simulink model "ARSinit"  (Simulink 6.6)
settings: Solver=ode1  SolverMode=SingleTasking  StartTime=0.0  StopTime=Tsim  FixedStep=0.001  RelTol=1e-3
PreLoadFcn:
  | load ARSdata
values from neighbouring files (symbols this model uses):
  car =     [ARSdata.mat]
  K = 0.025    [ARSdata.mat]
  meled_den = [1 -0.980198019802]    [ARSdata.mat]
  meled_num = [0.0049504950495 0.0049504950495]    [ARSdata.mat]
  mmecd_den = [1 -1]    [ARSdata.mat]
  mmecd_num = [0.05 0.05]    [ARSdata.mat]
  phid_den = [1 -1]    [ARSdata.mat]
  phid_num = [0.0005 0.0005]    [ARSdata.mat]
  scrtd_den = [1 -0.818181818182]    [ARSdata.mat]
  scrtd_num = [0.0181818181818 0.0181818181818]    [ARSdata.mat]
  sspeedd_den = [1 -0.818181818182]    [ARSdata.mat]
  sspeedd_num = [0.00909090909091 0.00909090909091]    [ARSdata.mat]
  vconvd_den = [1 -0.818181818182]    [ARSdata.mat]
  vconvd_num = [0.0909090909091 0.0909090909091]    [ARSdata.mat]
undefined symbols (not defined in the file or in its folder): sigbuilder_block
libraries: cstblocks x1
CloseFcn:
  | rtwprivate ssgencode ModelCloseRequest ARSinit
settings Model: Creator=Magna Steyr and PreeTec  LastModifiedBy=derler  ExtModeAutoUpdateStatusClock=off
settings OptimizationCC: InlineInvariantSignals=on  OptimizeModelRefInitCode=on  LifeSpan=1
settings DebuggingCC: SignalResolutionControl=TryResolveAllWithWarning  MultiTaskDSMMsg=warning  MultiTaskCondExecSysMsg=none  StrictBusMsg=None
settings RTWCC: SystemTargetFile=ert.tlc  GenCodeOnly=on  TemplateMakefile=ert_default_tmf  Description=RTW Embedded Coder (no auto configuration)  ProcessScript=ert_make_rtw_hook  IncludeERTFirstTime=on
settings CodeAppCC: IgnoreCustomStorageClasses=off
settings ERTTargetCC: TargetFcnLib=ansi_tfl_tmw.mat  GenFloatMathFcnCalls=ANSI_C  GenerateSampleERTMain=on  SupportContinuousTime=on  SupportNonInlinedSFcns=on  InlinedParameterPlacement=NonHierarchical  ERTCustomFileTemplate=example_file_process.tlc

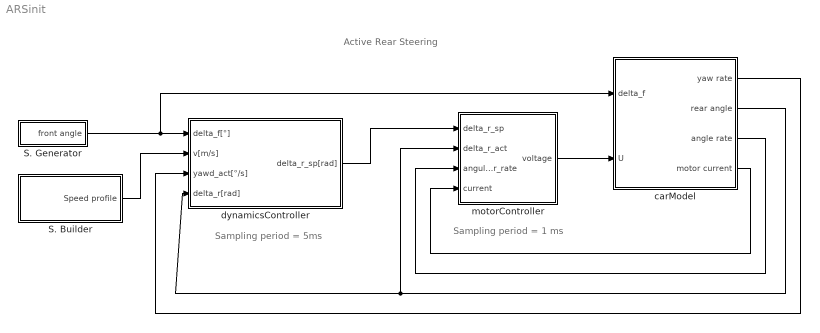
== system ARSinit ==
  note: Sampling period = 5ms
  note: Sampling period = 1 ms
  note: Active Rear Steering
  S. Builder : Subsystem  Tag=STV Subsys  LoadFcn=sigbuilder_block('load',[207 158.25 519.75 399.75 ]);  StartFcn=sigbuilder_block('start');  StopFcn=sigbuilder_block('stop');  ClipboardFcn=sigbuilder_block('clipboard');  mask(Sigbuilder block){}
      mask help: Sigbuilder GUI
      mask init:
      | if ~strcmp(get_param(bdroot(gcbh),'SimulationStatus'),'stopped') tuvar = sigbuilder_block('maskInit'); end
      settings: CopyFcn=sigbuilder_block('copy');  DeleteFcn=sigbuilder_block('delete');  ModelCloseFcn=sigbuilder_block('modelClose');  PreSaveFcn=sigbuilder_block('preSave');  NameChangeFcn=sigbuilder_block('namechange');  OpenFcn=sigbuilder_block('open',[207 158.25 519.75 399.75 ]);  CloseFcn=sigbuilder_block('close');
      mask Display: plot(0,0,100,100,[10,10,40,40,10],[80,20,20,80,80],[40,10],[50,50], [40,27,10],[65,72,56],[40,25,25,10],[28,28,43,43]);
  S. Generator : Subsystem
  carModel : Subsystem  TreatAsAtomicUnit=on  SystemSampleTime=0.001  RTWFcnName=carModel
      settings: RTWSystemCode=Function  RTWFcnNameOpts=User specified  RTWFileNameOpts=Use function name
  dynamicsController : Subsystem  TreatAsAtomicUnit=on  SystemSampleTime=0.005  RTWFcnName=dynamicsController
      settings: RTWSystemCode=Function  RTWFcnNameOpts=User specified  RTWFileNameOpts=Use function name
  motorController : Subsystem  TreatAsAtomicUnit=on  SystemSampleTime=0.001  RTWFcnName=motorController
      settings: RTWSystemCode=Function  RTWFcnNameOpts=User specified  RTWFileNameOpts=Use function name
  wires:
  S. Generator/1(front angle) -> dynamicsController/1(delta_f[°]), carModel/1(delta_f)
  S. Builder/1(Speed profile) -> dynamicsController/2(v[m/s])
  carModel/4(motor current) -> motorController/4(current)
  carModel/3(angle rate) -> motorController/3(angular_rate)
  carModel/2(rear angle) -> motorController/2(delta_r_act), dynamicsController/4(delta_r[rad])
  motorController/1(voltage) -> carModel/2(U)
  dynamicsController/1(delta_r_sp[rad]) -> motorController/1(delta_r_sp)
  carModel/1(yaw rate) -> dynamicsController/3(yawd_act[°/s])

== system ARSinit/S. Builder ==
  Demux : Demux  Tag=STV Demux  Outputs=1
  FromWs : FromWorkspace  Tag=STV FromWs  VariableName=tuvar  SampleTime=0.001  OutputAfterFinalValue=Holding final value  SigBuilderData=DataTag0  VnvData=DataTag1
      SigBuilderData=|
      | channels.label = 'Speed profile'
      | channels.allXData = {[0 8 11 20]}
      | channels.allYData = {[1.4 1.4 13.4 13.4]}
      | dataSet.timeRange = [0 20]
      | dataSet.name = 'Group 1'
  Speed profile : Outport  Tag=STV Outport
  wires:
  Demux/1 -> Speed profile/1
  FromWs/1 -> Demux/1

== system ARSinit/S. Generator ==
  Sum : Sum  Inputs=|++++
  smooth jump1 : Subsystem  AncestorBlock=joeslibrary/smooth jump  mask(Smooth jump){jump_time=6, minimum=-60, maximum=0, k=-10}
      mask prompts: jump_time "Jump time:"; minimum "Minimum value:"; maximum "Maximum value:"; k "Raise value:"
      mask help: x = scaling*tanh(clock-jump_time)
      mask Display: plot(-10:1:10,tanh(-10:1:10))
  smooth jump2 : Subsystem  AncestorBlock=joeslibrary/smooth jump  mask(Smooth jump){jump_time=1, minimum=0, maximum=60, k=10}
      mask prompts: jump_time "Jump time:"; minimum "Minimum value:"; maximum "Maximum value:"; k "Raise value:"
      mask help: x = scaling*tanh(clock-jump_time)
      mask Display: plot(-10:1:10,tanh(-10:1:10))
  smooth jump3 : Subsystem  AncestorBlock=joeslibrary/smooth jump  mask(Smooth jump){jump_time=12, minimum=0, maximum=20, k=10}
      mask prompts: jump_time "Jump time:"; minimum "Minimum value:"; maximum "Maximum value:"; k "Raise value:"
      mask help: x = scaling*tanh(clock-jump_time)
      mask Display: plot(-10:1:10,tanh(-10:1:10))
  smooth jump4 : Subsystem  AncestorBlock=joeslibrary/smooth jump  mask(Smooth jump){jump_time=17, minimum=-20, maximum=0, k=-10}
      mask prompts: jump_time "Jump time:"; minimum "Minimum value:"; maximum "Maximum value:"; k "Raise value:"
      mask help: x = scaling*tanh(clock-jump_time)
      mask Display: plot(-10:1:10,tanh(-10:1:10))
  front angle : Outport
  wires:
  smooth jump1/1(Out1) -> Sum/1
  smooth jump3/1(Out1) -> Sum/3
  smooth jump4/1(Out1) -> Sum/4
  smooth jump2/1(Out1) -> Sum/2
  Sum/1 -> front angle/1

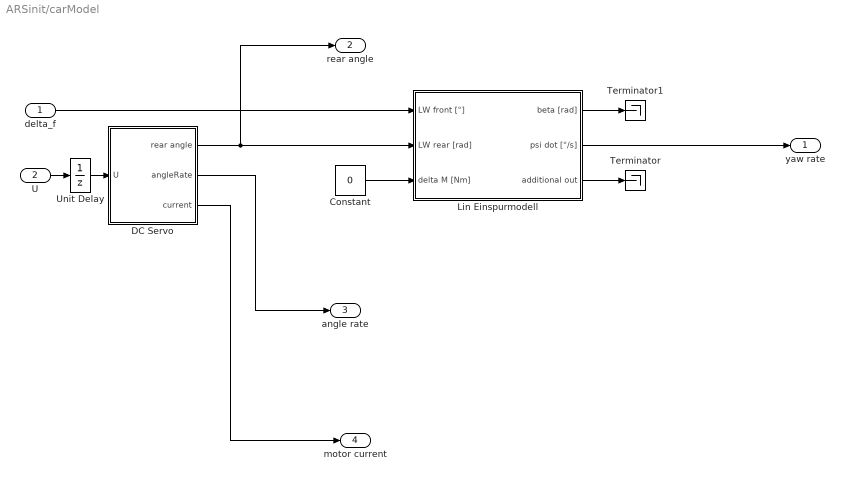
== system ARSinit/carModel ==
  delta_f : Inport
  U : Inport  Port=2
  Constant : Constant  Value=0
  DC Servo : Subsystem
  Lin Einspurmodell : Subsystem  AncestorBlock=joeslibrary/carspecific/Lin Einspurmodell  mask{car=car}
      mask prompts: car "car definition"
  Terminator : Terminator
  Terminator1 : Terminator
  Unit Delay : UnitDelay  SampleTime=-1
  yaw rate : Outport
  rear angle : Outport  Port=2
  angle rate : Outport  Port=3
  motor current : Outport  Port=4
  wires:
  Unit Delay/1 -> DC Servo/1(U)
  DC Servo/1(rear angle) -> Lin Einspurmodell/2(LW rear [rad]), rear angle/1
  DC Servo/3(current) -> motor current/1
  DC Servo/2(angleRate) -> angle rate/1
  U/1 -> Unit Delay/1
  Lin Einspurmodell/2(psi dot [°/s]) -> yaw rate/1
  delta_f/1 -> Lin Einspurmodell/1(LW front [°])
  Lin Einspurmodell/3(additional out) -> Terminator/1
  Lin Einspurmodell/1(beta [rad]) -> Terminator1/1
  Constant/1 -> Lin Einspurmodell/3(delta M [Nm])

== system ARSinit/dynamicsController ==
  delta_f[°] : Inport
  v[m/s] : Inport  Port=2
  yawd_act[°/s] : Inport  Port=3
  delta_r[rad] : Inport  Port=4
  Regler : Subsystem
  sollwertberechnung : Subsystem
  delta_r_sp[rad] : Outport
  wires:
  sollwertberechnung/1(psi_dot_soll [°/s]) -> Regler/3(psid_soll [°/s])
  v[m/s]/1 -> sollwertberechnung/2(v [m/s]), Regler/2(v [m/s])
  yawd_act[°/s]/1 -> Regler/4(psid_ist [°/s])
  delta_f[°]/1 -> sollwertberechnung/1(delta_v [°]), Regler/1(lrw [°])
  Regler/1(delta_h_soll [rad]) -> delta_r_sp[rad]/1
  delta_r[rad]/1 -> sollwertberechnung/3(delta_h [rad])

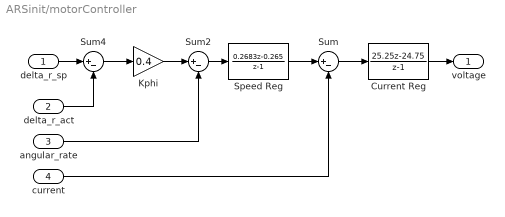
== system ARSinit/motorController ==
  delta_r_sp : Inport
  delta_r_act : Inport  Port=2
  angular_rate : Inport  Port=3
  current : Inport  Port=4
  Current Reg : DiscreteTransferFcn  Numerator=[25.25 -24.75]  Denominator=[1 -1]  SampleTime=-1
  Kphi : Gain  Gain=0.4
  Speed Reg : DiscreteTransferFcn  Numerator=[0.2683 -0.265]  Denominator=[1 -1]  SampleTime=-1
  Sum : Sum  Inputs=|+-
  Sum2 : Sum  Inputs=|+-
  Sum4 : Sum  Inputs=|+-
  voltage : Outport
  wires:
  Sum/1 -> Current Reg/1
  Sum2/1 -> Speed Reg/1
  Speed Reg/1 -> Sum/1
  Kphi/1 -> Sum2/1
  Sum4/1 -> Kphi/1
  Current Reg/1 -> voltage/1
  delta_r_sp/1 -> Sum4/1
  current/1 -> Sum/2
  angular_rate/1 -> Sum2/2
  delta_r_act/1 -> Sum4/2

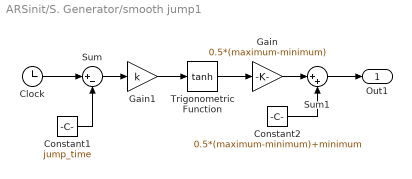
== system ARSinit/S. Generator/smooth jump1 ==
  Clock : Clock
      settings: Decimation=10
  Constant1 : Constant  Value=jump_time
  Constant2 : Constant  Value=0.5*(maximum-minimum)+minimum
  Gain : Gain  Gain=0.5*(maximum-minimum)  SaturateOnIntegerOverflow=on
  Gain1 : Gain  Gain=k  SaturateOnIntegerOverflow=on
  Sum : Sum  Inputs=|+-  SaturateOnIntegerOverflow=on
  Sum1 : Sum  Inputs=|++  SaturateOnIntegerOverflow=on
  Trigonometric Function : Trigonometry  Operator=tanh  OutputSignalType=real
  Out1 : Outport
  wires:
  Sum/1 -> Gain1/1
  Clock/1 -> Sum/1
  Constant1/1 -> Sum/2
  Trigonometric Function/1 -> Gain/1
  Gain/1 -> Sum1/1
  Sum1/1 -> Out1/1
  Constant2/1 -> Sum1/2
  Gain1/1 -> Trigonometric Function/1

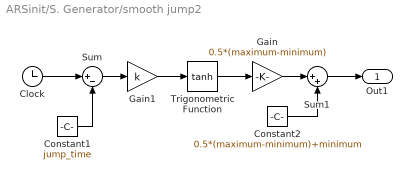
== system ARSinit/S. Generator/smooth jump2 ==
  Clock : Clock
      settings: Decimation=10
  Constant1 : Constant  Value=jump_time
  Constant2 : Constant  Value=0.5*(maximum-minimum)+minimum
  Gain : Gain  Gain=0.5*(maximum-minimum)  SaturateOnIntegerOverflow=on
  Gain1 : Gain  Gain=k  SaturateOnIntegerOverflow=on
  Sum : Sum  Inputs=|+-  SaturateOnIntegerOverflow=on
  Sum1 : Sum  Inputs=|++  SaturateOnIntegerOverflow=on
  Trigonometric Function : Trigonometry  Operator=tanh  OutputSignalType=real
  Out1 : Outport
  wires:
  Sum/1 -> Gain1/1
  Clock/1 -> Sum/1
  Constant1/1 -> Sum/2
  Trigonometric Function/1 -> Gain/1
  Gain/1 -> Sum1/1
  Sum1/1 -> Out1/1
  Constant2/1 -> Sum1/2
  Gain1/1 -> Trigonometric Function/1

== system ARSinit/S. Generator/smooth jump3 ==
  Clock : Clock
      settings: Decimation=10
  Constant1 : Constant  Value=jump_time
  Constant2 : Constant  Value=0.5*(maximum-minimum)+minimum
  Gain : Gain  Gain=0.5*(maximum-minimum)  SaturateOnIntegerOverflow=on
  Gain1 : Gain  Gain=k  SaturateOnIntegerOverflow=on
  Sum : Sum  Inputs=|+-  SaturateOnIntegerOverflow=on
  Sum1 : Sum  Inputs=|++  SaturateOnIntegerOverflow=on
  Trigonometric Function : Trigonometry  Operator=tanh  OutputSignalType=real
  Out1 : Outport
  wires:
  Gain1/1 -> Trigonometric Function/1
  Constant2/1 -> Sum1/2
  Sum1/1 -> Out1/1
  Gain/1 -> Sum1/1
  Trigonometric Function/1 -> Gain/1
  Constant1/1 -> Sum/2
  Clock/1 -> Sum/1
  Sum/1 -> Gain1/1

== system ARSinit/S. Generator/smooth jump4 ==
  Clock : Clock
      settings: Decimation=10
  Constant1 : Constant  Value=jump_time
  Constant2 : Constant  Value=0.5*(maximum-minimum)+minimum
  Gain : Gain  Gain=0.5*(maximum-minimum)  SaturateOnIntegerOverflow=on
  Gain1 : Gain  Gain=k  SaturateOnIntegerOverflow=on
  Sum : Sum  Inputs=|+-  SaturateOnIntegerOverflow=on
  Sum1 : Sum  Inputs=|++  SaturateOnIntegerOverflow=on
  Trigonometric Function : Trigonometry  Operator=tanh  OutputSignalType=real
  Out1 : Outport
  wires:
  Gain1/1 -> Trigonometric Function/1
  Constant2/1 -> Sum1/2
  Sum1/1 -> Out1/1
  Gain/1 -> Sum1/1
  Trigonometric Function/1 -> Gain/1
  Constant1/1 -> Sum/2
  Clock/1 -> Sum/1
  Sum/1 -> Gain1/1

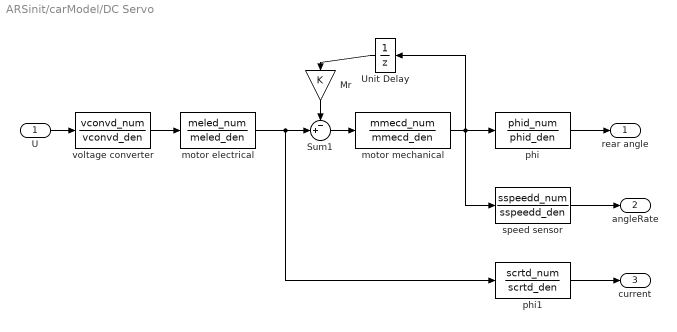
== system ARSinit/carModel/DC Servo ==
  U : Inport
  Mr : Gain  Orientation=down  Gain=K
  Sum1 : Sum  Inputs=-+|
  Unit Delay : UnitDelay  Orientation=left  SampleTime=-1
  motor electrical : DiscreteTransferFcn  Numerator=meled_num  Denominator=meled_den  SampleTime=-1
  motor mechanical : DiscreteTransferFcn  Numerator=mmecd_num  Denominator=mmecd_den  SampleTime=-1
  phi : DiscreteTransferFcn  Numerator=phid_num  Denominator=phid_den  SampleTime=-1
  phi1 : DiscreteTransferFcn  Numerator=scrtd_num  Denominator=scrtd_den  SampleTime=-1
  speed sensor : DiscreteTransferFcn  Numerator=sspeedd_num  Denominator=sspeedd_den  SampleTime=-1
  voltage converter : DiscreteTransferFcn  Numerator=vconvd_num  Denominator=vconvd_den  SampleTime=-1
  rear angle : Outport
  angleRate : Outport  Port=2
  current : Outport  Port=3
  wires:
  Unit Delay/1 -> Mr/1
  motor mechanical/1 -> speed sensor/1, Unit Delay/1, phi/1
  Sum1/1 -> motor mechanical/1
  Mr/1 -> Sum1/1
  motor electrical/1 -> phi1/1, Sum1/2
  voltage converter/1 -> motor electrical/1
  phi/1 -> rear angle/1
  U/1 -> voltage converter/1
  phi1/1 -> current/1
  speed sensor/1 -> angleRate/1

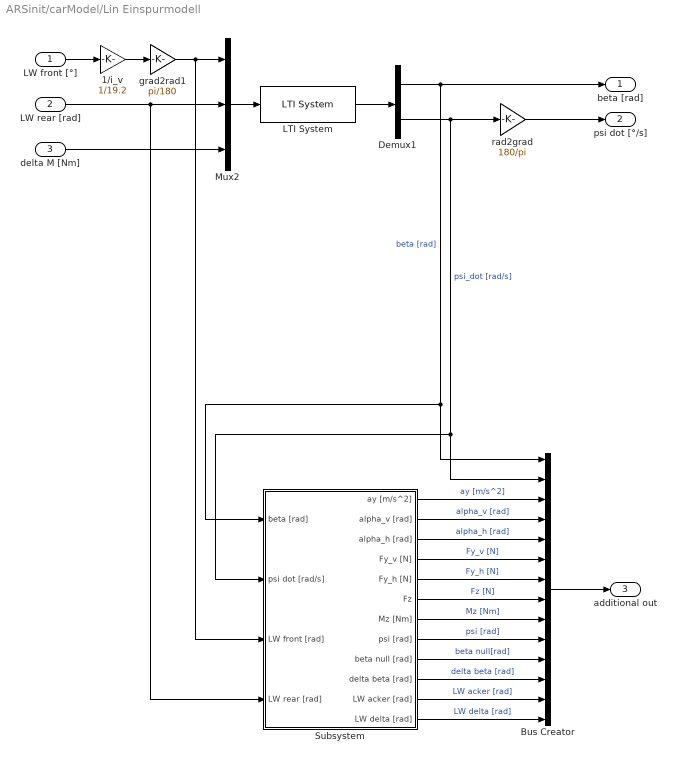
== system ARSinit/carModel/Lin Einspurmodell ==
  LW front [°] : Inport
  LW rear [rad] : Inport  Port=2
  delta M [Nm] : Inport  Port=3
  1/i_v : Gain  Gain=1/19.2  SaturateOnIntegerOverflow=on
  Bus Creator : BusCreator  Inputs=14
  Demux1 : Demux  Outputs=2
  LTI System : cstblocks/LTI System  SystemSampleTime=-1  sys=carLTI  IC=[]
  Mux2 : Mux  Inputs=3
  Subsystem : Subsystem
  grad2rad1 : Gain  Gain=pi/180  SaturateOnIntegerOverflow=on
  rad2grad : Gain  Gain=180/pi  SaturateOnIntegerOverflow=on
  beta [rad] : Outport
  psi dot [°/s] : Outport  Port=2
  additional out : Outport  Port=3
  wires:
  LTI System/1 -> Demux1/1
  Mux2/1 -> LTI System/1
  Demux1/2 -> Subsystem/2(psi dot [rad/s]), Bus Creator/2, rad2grad/1  "psi_dot [rad/s]"
  LW rear [rad]/1 -> Mux2/2, Subsystem/4(LW rear [rad])
  Demux1/1 -> beta [rad]/1, Subsystem/1(beta [rad]), Bus Creator/1  "beta [rad]"
  delta M [Nm]/1 -> Mux2/3
  Subsystem/1(ay [m/s^2]) -> Bus Creator/3  "ay [m/s^2]"
  Bus Creator/1 -> additional out/1
  Subsystem/2(alpha_v [rad]) -> Bus Creator/4  "alpha_v [rad]"
  Subsystem/3(alpha_h [rad]) -> Bus Creator/5  "alpha_h [rad]"
  Subsystem/4(Fy_v [N]) -> Bus Creator/6  "Fy_v [N]"
  Subsystem/5(Fy_h [N]) -> Bus Creator/7  "Fy_h [N]"
  Subsystem/6(Fz) -> Bus Creator/8  "Fz [N]"
  Subsystem/7(Mz [Nm]) -> Bus Creator/9  "Mz [Nm]"
  Subsystem/8(psi [rad]) -> Bus Creator/10  "psi [rad]"
  Subsystem/9(beta null [rad]) -> Bus Creator/11  "beta null[rad]"
  Subsystem/10(delta beta [rad]) -> Bus Creator/12  "delta beta [rad]"
  Subsystem/11(LW acker [rad]) -> Bus Creator/13  "LW acker [rad]"
  Subsystem/12(LW delta [rad]) -> Bus Creator/14  "LW delta [rad]"
  LW front [°]/1 -> 1/i_v/1
  grad2rad1/1 -> Mux2/1, Subsystem/3(LW front [rad])
  1/i_v/1 -> grad2rad1/1
  rad2grad/1 -> psi dot [°/s]/1

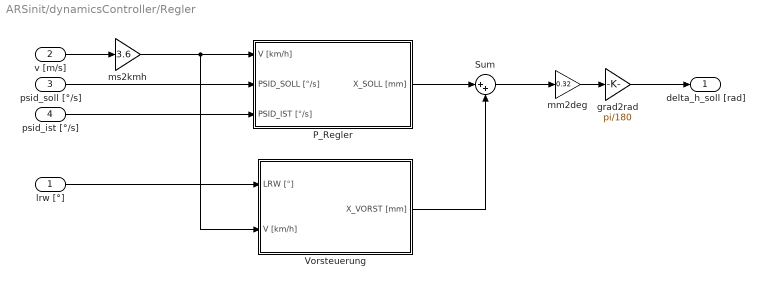
== system ARSinit/dynamicsController/Regler ==
  lrw [°] : Inport
  v [m/s] : Inport  Port=2
  psid_soll [°/s] : Inport  Port=3
  psid_ist [°/s] : Inport  Port=4
  P_Regler : Subsystem
  Sum : Sum  Inputs=|++  SaturateOnIntegerOverflow=on
  Vorsteuerung : Subsystem
  grad2rad : Gain  Gain=pi/180  SaturateOnIntegerOverflow=on
  mm2deg : Gain  Gain=0.32  SaturateOnIntegerOverflow=on
  ms2kmh : Gain  Gain=3.6  SaturateOnIntegerOverflow=on
  delta_h_soll [rad] : Outport
  wires:
  v [m/s]/1 -> ms2kmh/1
  psid_soll [°/s]/1 -> P_Regler/2(PSID_SOLL [°/s])
  P_Regler/1(X_SOLL [mm]) -> Sum/1
  psid_ist [°/s]/1 -> P_Regler/3(PSID_IST [°/s])
  Vorsteuerung/1(X_VORST [mm]) -> Sum/2
  lrw [°]/1 -> Vorsteuerung/1(LRW [°])
  mm2deg/1 -> grad2rad/1
  grad2rad/1 -> delta_h_soll [rad]/1
  Sum/1 -> mm2deg/1
  ms2kmh/1 -> P_Regler/1(V [km/h]), Vorsteuerung/2(V [km/h])

== system ARSinit/dynamicsController/sollwertberechnung ==
  delta_v [°] : Inport
  v [m/s] : Inport  Port=2
  delta_h [rad] : Inport  Port=3
  1/i_v : Gain  Gain=1/19.2  SaturateOnIntegerOverflow=on
  Gain2 : Gain  Gain=180/pi  SaturateOnIntegerOverflow=on
  ay_estimate : Subsystem
  grad2rad1 : Gain  Gain=pi/180  SaturateOnIntegerOverflow=on
  psi_dot_soll [°/s] : Outport
  wires:
  Gain2/1 -> psi_dot_soll [°/s]/1
  v [m/s]/1 -> ay_estimate/1(v)
  delta_h [rad]/1 -> ay_estimate/3(delta_h)
  ay_estimate/1(psi_dot) -> Gain2/1
  1/i_v/1 -> grad2rad1/1
  grad2rad1/1 -> ay_estimate/2(delta_v)
  delta_v [°]/1 -> 1/i_v/1

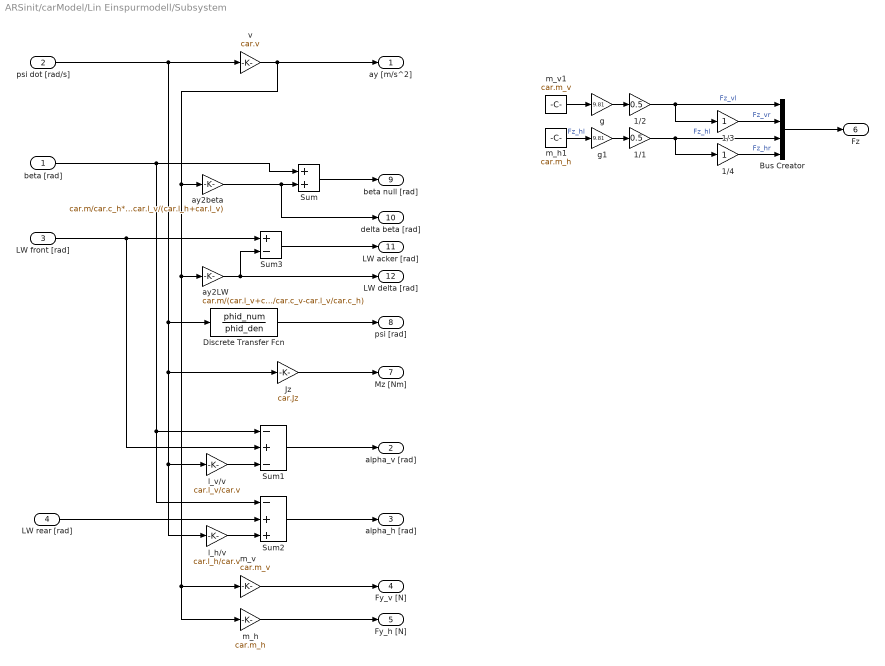
== system ARSinit/carModel/Lin Einspurmodell/Subsystem ==
  beta [rad] : Inport
  psi dot [rad/s] : Inport  Port=2
  LW front [rad] : Inport  Port=3
  LW rear [rad] : Inport  Port=4
  1/1 : Gain  Gain=0.5  SaturateOnIntegerOverflow=on
  1/2 : Gain  Gain=0.5  SaturateOnIntegerOverflow=on
  1/3 : Gain  SaturateOnIntegerOverflow=on
  1/4 : Gain  SaturateOnIntegerOverflow=on
  Bus Creator : BusCreator
  Discrete Transfer Fcn : DiscreteTransferFcn  Numerator=phid_num  Denominator=phid_den  SampleTime=-1
  Jz : Gain  Gain=car.Jz  SaturateOnIntegerOverflow=on
  Sum : Sum  SaturateOnIntegerOverflow=on
  Sum1 : Sum  Inputs=-+-  SaturateOnIntegerOverflow=on
  Sum2 : Sum  Inputs=-++  SaturateOnIntegerOverflow=on
  Sum3 : Sum  Inputs=+-  SaturateOnIntegerOverflow=on
  ay2LW : Gain  Gain=car.m/(car.l_v+car.l_h)*(car.l_h/car.c_v-car.l_v/car.c_h)  SaturateOnIntegerOverflow=on
  ay2beta : Gain  Gain=car.m/car.c_h*car.l_v/(car.l_h+car.l_v)  SaturateOnIntegerOverflow=on
  g : Gain  Gain=9.81  SaturateOnIntegerOverflow=on
  g1 : Gain  Gain=9.81  SaturateOnIntegerOverflow=on
  l_h/v : Gain  Gain=car.l_h/car.v  SaturateOnIntegerOverflow=on
  l_v/v : Gain  Gain=car.l_v/car.v  SaturateOnIntegerOverflow=on
  m_h : Gain  Gain=car.m_h  SaturateOnIntegerOverflow=on
  m_h1 : Constant  Value=car.m_h
  m_v : Gain  Gain=car.m_v  SaturateOnIntegerOverflow=on
  m_v1 : Constant  Value=car.m_v
  v : Gain  Gain=car.v  SaturateOnIntegerOverflow=on
  ay [m/s^2] : Outport
  alpha_v [rad] : Outport  Port=2
  alpha_h [rad] : Outport  Port=3
  Fy_v [N] : Outport  Port=4
  Fy_h [N] : Outport  Port=5
  Fz : Outport  Port=6
  Mz [Nm] : Outport  Port=7
  psi [rad] : Outport  Port=8
  beta null [rad] : Outport  Port=9
  delta beta [rad] : Outport  Port=10
  LW acker [rad] : Outport  Port=11
  LW delta [rad] : Outport  Port=12
  wires:
  Sum/1 -> beta null [rad]/1
  Discrete Transfer Fcn/1 -> psi [rad]/1
  Jz/1 -> Mz [Nm]/1
  Sum3/1 -> LW acker [rad]/1
  Sum2/1 -> alpha_h [rad]/1
  l_h/v/1 -> Sum2/3
  Sum1/1 -> alpha_v [rad]/1
  l_v/v/1 -> Sum1/3
  ay2LW/1 -> LW delta [rad]/1, Sum3/2
  ay2beta/1 -> Sum/2, delta beta [rad]/1
  v/1 -> ay [m/s^2]/1, ay2beta/1, ay2LW/1, m_v/1, m_h/1
  psi dot [rad/s]/1 -> v/1, Discrete Transfer Fcn/1, Jz/1, l_v/v/1, l_h/v/1
  beta [rad]/1 -> Sum/1, Sum1/1, Sum2/1
  LW front [rad]/1 -> Sum1/2, Sum3/1
  LW rear [rad]/1 -> Sum2/2
  m_v/1 -> Fy_v [N]/1
  m_h/1 -> Fy_h [N]/1
  Bus Creator/1 -> Fz/1
  m_h1/1 -> g1/1  "Fz_hl"
  g/1 -> 1/2/1
  m_v1/1 -> g/1
  1/2/1 -> Bus Creator/1, 1/3/1  "Fz_vl"
  g1/1 -> 1/1/1
  1/1/1 -> Bus Creator/3, 1/4/1  "Fz_hl"
  1/3/1 -> Bus Creator/2  "Fz_vr"
  1/4/1 -> Bus Creator/4  "Fz_hr"

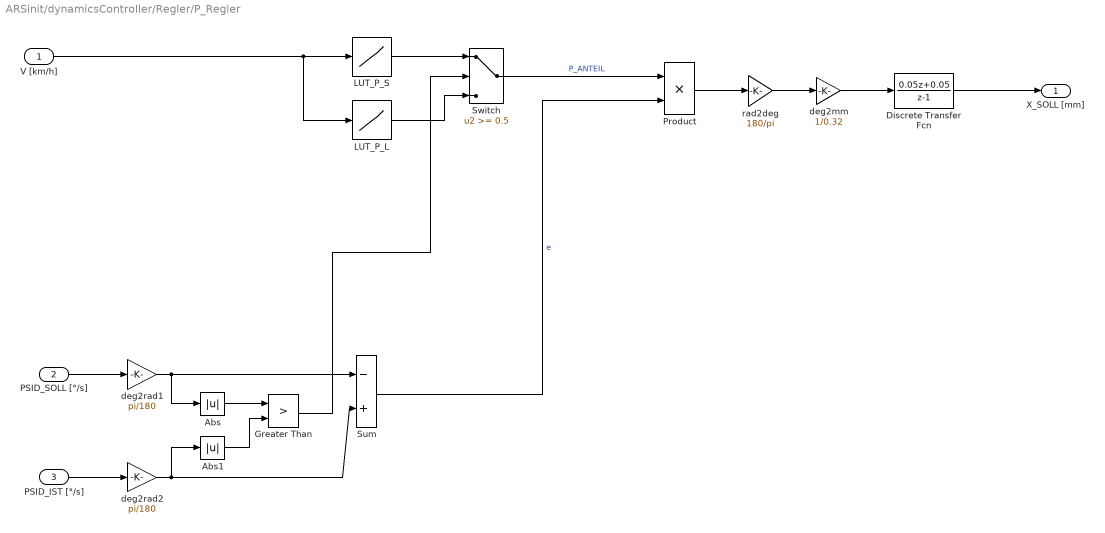
== system ARSinit/dynamicsController/Regler/P_Regler ==
  V [km/h] : Inport
  PSID_SOLL [°/s] : Inport  Port=2
  PSID_IST [°/s] : Inport  Port=3
  Abs : Abs  SaturateOnIntegerOverflow=on
  Abs1 : Abs  SaturateOnIntegerOverflow=on
  Discrete Transfer Fcn : DiscreteTransferFcn  Numerator=[0.05 0.05]  Denominator=[1 -1]  SampleTime=-1
  Greater Than : RelationalOperator  Operator=>  LogicOutDataTypeMode=Boolean  ZeroCross=off
  LUT_P_L : Lookup  InputValues="[40  50    100   200]"  OutputValues="[0  0.04  0.04  0.04]"  LookUpMeth=Interpolation-Use End Values  OutDataTypeMode=double  OutScaling=2^-10  RndMeth=Nearest
  LUT_P_S : Lookup  InputValues="[40  50    100   200]"  OutputValues="[0  0.004  0.004  0.004]"  LookUpMeth=Interpolation-Use End Values  OutDataTypeMode=double  OutScaling=2^-10  RndMeth=Nearest
  Product : Product  SaturateOnIntegerOverflow=on
  Sum : Sum  Inputs=-+  SaturateOnIntegerOverflow=on
  Switch : Switch  Threshold=0.5  SaturateOnIntegerOverflow=on
  deg2mm : Gain  Gain=1/0.32  SaturateOnIntegerOverflow=on
  deg2rad1 : Gain  Gain=pi/180  SaturateOnIntegerOverflow=on
  deg2rad2 : Gain  Gain=pi/180  SaturateOnIntegerOverflow=on
  rad2deg : Gain  Gain=180/pi  SaturateOnIntegerOverflow=on
  X_SOLL [mm] : Outport
  wires:
  Greater Than/1 -> Switch/2
  rad2deg/1 -> deg2mm/1
  V [km/h]/1 -> LUT_P_L/1, LUT_P_S/1
  Abs/1 -> Greater Than/1
  Abs1/1 -> Greater Than/2
  PSID_SOLL [°/s]/1 -> deg2rad1/1
  PSID_IST [°/s]/1 -> deg2rad2/1
  LUT_P_S/1 -> Switch/1
  LUT_P_L/1 -> Switch/3
  Switch/1 -> Product/1  "P_ANTEIL"
  Sum/1 -> Product/2  "e"
  Product/1 -> rad2deg/1
  deg2rad1/1 -> Abs/1, Sum/1
  deg2rad2/1 -> Abs1/1, Sum/2
  deg2mm/1 -> Discrete Transfer Fcn/1
  Discrete Transfer Fcn/1 -> X_SOLL [mm]/1

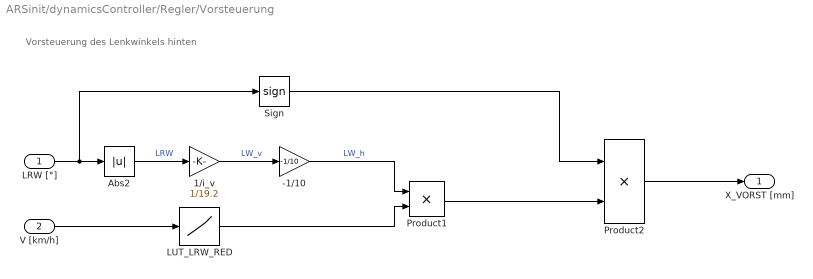
== system ARSinit/dynamicsController/Regler/Vorsteuerung ==
  note: Vorsteuerung des Lenkwinkels hinten
  LRW [°] : Inport
  V [km/h] : Inport  Port=2
  -1/10 : Gain  Gain=-1/10  SaturateOnIntegerOverflow=on
  1/i_v : Gain  Gain=1/19.2  SaturateOnIntegerOverflow=on
  Abs2 : Abs  SaturateOnIntegerOverflow=on
  LUT_LRW_RED : Lookup  InputValues=[0 10 40]  OutputValues=[1 1 0]  LookUpMeth=Interpolation-Use End Values  RndMeth=Nearest  SaturateOnIntegerOverflow=on
  Product1 : Product  SaturateOnIntegerOverflow=on
  Product2 : Product  SaturateOnIntegerOverflow=on
  Sign : Signum
  X_VORST [mm] : Outport
  wires:
  LUT_LRW_RED/1 -> Product1/2
  Product1/1 -> Product2/2
  Abs2/1 -> 1/i_v/1  "LRW"
  V [km/h]/1 -> LUT_LRW_RED/1
  Product2/1 -> X_VORST [mm]/1
  Sign/1 -> Product2/1
  LRW [°]/1 -> Abs2/1, Sign/1
  1/i_v/1 -> -1/10/1  "LW_v"
  -1/10/1 -> Product1/1  "LW_h"

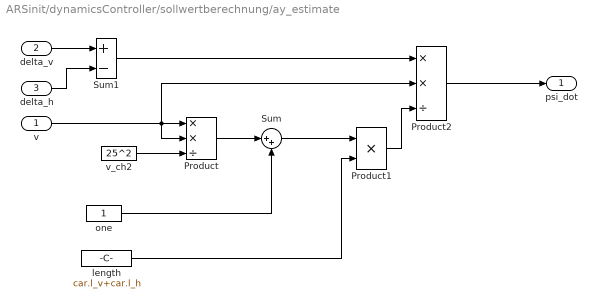
== system ARSinit/dynamicsController/sollwertberechnung/ay_estimate ==
  v : Inport
  delta_v : Inport  Port=2
  delta_h : Inport  Port=3
  Product : Product  Inputs=**/  SaturateOnIntegerOverflow=on
  Product1 : Product  SaturateOnIntegerOverflow=on
  Product2 : Product  Inputs=**/  SaturateOnIntegerOverflow=on
  Sum : Sum  Inputs=|++  SaturateOnIntegerOverflow=on
  Sum1 : Sum  Inputs=+-  SaturateOnIntegerOverflow=on
  length : Constant  Value=car.l_v+car.l_h
  one : Constant
  v_ch2 : Constant  Value=25^2
  psi_dot : Outport
  wires:
  Sum1/1 -> Product2/1
  delta_h/1 -> Sum1/2
  delta_v/1 -> Sum1/1
  v_ch2/1 -> Product/3
  Product2/1 -> psi_dot/1
  Product1/1 -> Product2/3
  length/1 -> Product1/2
  Sum/1 -> Product1/1
  one/1 -> Sum/2
  Product/1 -> Sum/1
  v/1 -> Product/2, Product2/2, Product/1
